simulink model "iterative_elastic"  (R2022a)
settings: Solver=VariableStepAuto  StartTime=0.0  StopTime=30  RelTol=1e-3
undefined symbols (not defined in the file): Kd, Kp, qd
libraries: simulink x1, simulink_extras x1
settings Model: Creator=fabioscap  LastModifiedBy=dennis
settings DebuggingCC: UnconnectedInputMsg=warning  UnconnectedOutputMsg=warning  UnconnectedLineMsg=warning
settings RTWCC: DLArmComputeVersion=19.05

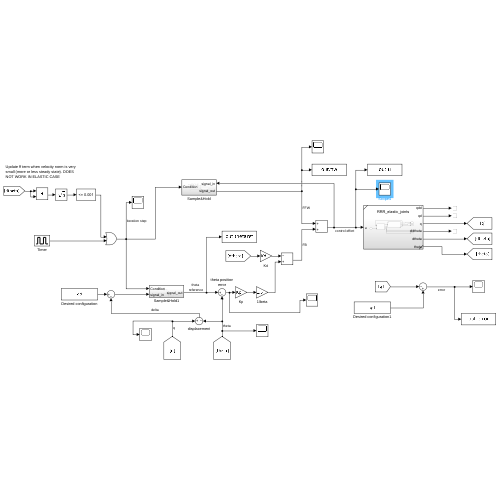
[thumbnail: Simulink's stored preview of the top-level diagram]
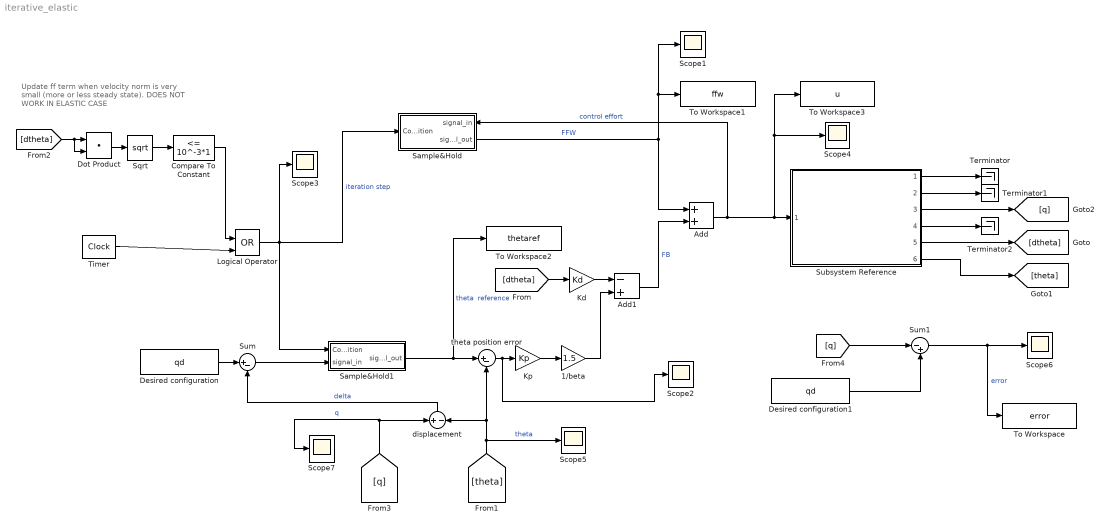
== system iterative_elastic ==
  note: Update ff term when velocity norm is very small (more or less steady state). DOES NOT WORK IN ELASTIC CASE
  1/beta : Gain  Gain=1.5
  Add : Sum
  Add1 : Sum  Inputs=-+
  Compare To Constant : simulink/Logic and Bit Operations/Compare To Constant  relop=<=  const=10^-3*1  OutDataTypeStr=boolean
  Desired configuration : Constant  Value=qd
  Desired configuration1 : Constant  Value=qd
  Dot Product : DotProduct  OutDataTypeStr=Inherit: Inherit via internal rule
  Kd : Gain  Gain=Kd
  Kp : Gain  Gain=Kp
  Logical Operator : Logic  Operator=OR  IconShape=distinctive  AllPortsSameDT=off  OutDataTypeStr=boolean
  Sample&Hold : Subsystem
      settings: PortSchema="{\"entries\":[{\"content\":{\"sides\":[{\"content\":{\"connectorIds\":[\"In1\"]},\"type\":\"ConnectorPlacement.EquallySpacedRectSide\",\"uuid\":\"4e144169-49b5-4e4c-b5f4-9ef7c3f2f0f9\"},{\"content\":{\"connectorIds\":[\"In2\",\"Out1\"],\"side\":\"RIGHT\"},\"type\":\"ConnectorPlacement.EquallySpacedRectSide\",\"uuid\":\"f363b949-3911-4beb-ab4e-918606327600\"},{\"content\":{\"connectorIds\":[],\"side\":\"TOP\"},\"type\":\"ConnectorPlacement.EquallySpacedRectSide\",\"uuid\":\"9c880683-fb68-40e9-87c7-4f0e0baabf9f\"}]},\"type\":\"ConnectorPlacement.EquallySpacedConnector\",\"uuid\":\"d3c18749-4c54-4ed6-af1e-c9020595430a\"}],\"packageUris\":[\"http://schema.mathworks.com/mf0/Connector/R2020b\"],\"version\":\"1.0\"}"
  Sample&Hold1 : Subsystem
  Scope{1..7} (7 alike) : Scope
  Sqrt : Sqrt
  Subsystem Reference : Subsystem  ReferencedSubsystem=RRR_elastic_joints
  Sum : Sum  Inputs=|+-
  Sum1 : Sum  Inputs=|-+
  Terminator : Terminator
  Terminator1 : Terminator
  Terminator2 : Terminator
  Timer : simulink_extras/Flip Flops/Clock  period=4
  To Workspace : ToWorkspace  VariableName=error  SaveFormat=Timeseries  SampleTime=-1
  To Workspace1 : ToWorkspace  VariableName=ffw  SaveFormat=Timeseries  SampleTime=-1
  To Workspace2 : ToWorkspace  VariableName=thetaref  SaveFormat=Timeseries  SampleTime=-1
  To Workspace3 : ToWorkspace  VariableName=u  SaveFormat=Timeseries  SampleTime=-1
  displacement : Sum  Inputs=+-
  theta position error : Sum  Inputs=|+-
  wires:
  Sample&Hold/1(signal_out) -> Add/1, Scope1/1, To Workspace1/1  "FFW"
  Kd/1 -> Add1/1
  Add1/1 -> Add/2  "FB"
  1/beta/1 -> Add1/2
  [theta] -> Scope5/1, displacement/2, theta position error/2  "theta"
  Dot Product/1 -> Sqrt/1
  [dtheta] -> Kd/1
  Kp/1 -> 1/beta/1
  Sqrt/1 -> Compare To Constant/1
  Subsystem Reference/5 -> [dtheta]
  Subsystem Reference/6 -> [theta]
  [dtheta] -> Dot Product/2, Dot Product/1
  Subsystem Reference/3 -> [q]
  [q] -> Scope7/1, displacement/1  "q"
  Sample&Hold1/1(signal_out) -> theta position error/1, To Workspace2/1  "theta  reference"
  displacement/1 -> Sum/2  "delta"
  Sum/1 -> Sample&Hold1/2(signal_in)
  [q] -> Sum1/1
  Desired configuration1/1 -> Sum1/2
  Sum1/1 -> To Workspace/1, Scope6/1  "error"
  Subsystem Reference/1 -> Terminator/1
  Subsystem Reference/2 -> Terminator1/1
  Subsystem Reference/4 -> Terminator2/1
  Logical Operator/1 -> Sample&Hold/1(Condition), Sample&Hold1/1(Condition), Scope3/1  "iteration step"
  Desired configuration/1 -> Sum/1
  Timer/1 -> Logical Operator/2
  Compare To Constant/1 -> Logical Operator/1
  theta position error/1 -> Scope2/1, Kp/1
  Add/1 -> Sample&Hold/2(signal_in), Scope4/1, To Workspace3/1, Subsystem Reference/1  "control effort"

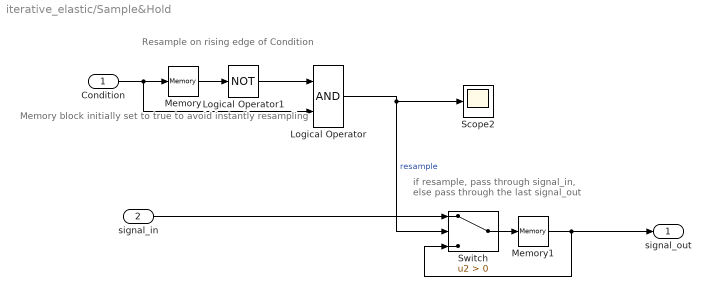
== system iterative_elastic/Sample&Hold ==
  note: Memory block initially set to true to avoid instantly resampling
  note: if resample, pass through signal_in,
      | else pass through the last signal_out
  note: Resample on rising edge of Condition
  Condition : Inport
  signal_in : Inport  Port=2
  Logical Operator : Logic  AllPortsSameDT=off  OutDataTypeStr=boolean
  Logical Operator1 : Logic  Operator=NOT  AllPortsSameDT=off  OutDataTypeStr=boolean
  Memory : Memory  InitialCondition=1
  Memory1 : Memory
  Scope2 : Scope
  Switch : Switch  Criteria=u2 > Threshold  SaturateOnIntegerOverflow=off  InputSameDT=off
  signal_out : Outport
  wires:
  Condition/1 -> Logical Operator/2, Memory/1
  Memory/1 -> Logical Operator1/1
  Logical Operator1/1 -> Logical Operator/1
  signal_in/1 -> Switch/1
  Logical Operator/1 -> Scope2/1, Switch/2  "resample"
  Memory1/1 -> Switch/3, signal_out/1
  Switch/1 -> Memory1/1

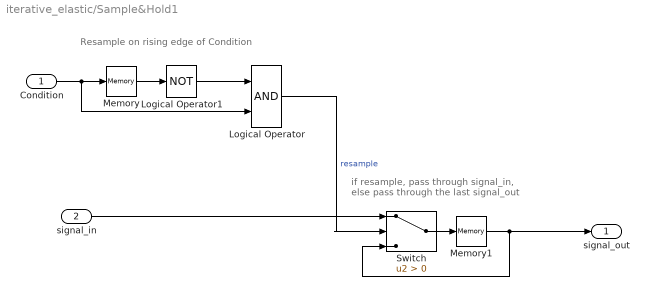
== system iterative_elastic/Sample&Hold1 ==
  note: if resample, pass through signal_in,
      | else pass through the last signal_out
  note: Resample on rising edge of Condition
  Condition : Inport
  signal_in : Inport  Port=2
  Logical Operator : Logic  AllPortsSameDT=off  OutDataTypeStr=boolean
  Logical Operator1 : Logic  Operator=NOT  AllPortsSameDT=off  OutDataTypeStr=boolean
  Memory : Memory  InitialCondition=1
  Memory1 : Memory  InitialCondition=qd
  Switch : Switch  Criteria=u2 > Threshold  SaturateOnIntegerOverflow=off  InputSameDT=off
  signal_out : Outport
  wires:
  Condition/1 -> Logical Operator/2, Memory/1
  Memory/1 -> Logical Operator1/1
  Logical Operator1/1 -> Logical Operator/1
  signal_in/1 -> Switch/1
  Logical Operator/1 -> Switch/2  "resample"
  Memory1/1 -> Switch/3, signal_out/1
  Switch/1 -> Memory1/1
